simulink library "actuator_meas_bus"  (R2018b)
settings: Solver=VariableStepAuto  StartTime=0.0  StopTime=10.0  RelTol=1e-3
undefined symbols (not defined in the file): mtq_power, mtq_valid, rwa_power, rwa_rpm, rwa_valid
settings Model: Creator=taylorreynolds  LastModifiedBy=taylorreynolds

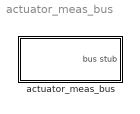
== system actuator_meas_bus ==
  actuator_meas_bus : Subsystem

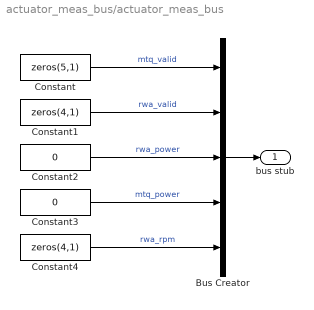
== system actuator_meas_bus/actuator_meas_bus ==
  Bus Creator : BusCreator  Inputs=mtq_valid,rwa_valid,rwa_power,mtq_power,rwa_rpm  OutDataTypeStr=Bus: actuator_meas
  Constant : Constant  Value=zeros(5,1)  OutDataTypeStr=boolean
  Constant1 : Constant  Value=zeros(4,1)  OutDataTypeStr=boolean
  Constant2 : Constant  Value=0  OutDataTypeStr=double
  Constant3 : Constant  Value=0  OutDataTypeStr=double
  Constant4 : Constant  Value=zeros(4,1)  OutDataTypeStr=double
  bus stub : Outport  OutDataTypeStr=Bus: actuator_meas
  wires:
  Bus Creator/1 -> bus stub/1
  Constant/1 -> Bus Creator/1  "mtq_valid"
  Constant1/1 -> Bus Creator/2  "rwa_valid"
  Constant2/1 -> Bus Creator/3  "rwa_power"
  Constant3/1 -> Bus Creator/4  "mtq_power"
  Constant4/1 -> Bus Creator/5  "rwa_rpm"
